simulink model "find6DOFSnellMin9_th"  (R2018b)
settings: Solver=ode8  StartTime=0.0  StopTime=length+1  FixedStep=1  RelTol=1e-3  EnableMultiTasking=on
StopFcn:
  | stopCallback
values from neighbouring files (symbols this model uses):
  botDot1 = zeros(length,2)    [find6DOFSnellMin9_ts.m]
  botDot2 = zeros(length,2)    [find6DOFSnellMin9_ts.m]
  botDot3 = zeros(length,2)    [find6DOFSnellMin9_ts.m]
libraries: find6DOFSnellMin9_cl x1
settings Model: SimulationMode=external  Creator=MAE-NCSUCORE  LastModifiedBy=MAE-NCSUCORE
settings SolverCC: ConcurrentTasks=on  AutoInsertRateTranBlk=on
settings DataIOCC: SaveFormat=StructureWithTime
settings OptimizationCC: BlockReduction=off  OptimizeBlockIOStorage=off  BufferReuse=off  GlobalBufferReuse=off  ExpressionFolding=off  LocalBlockOutputs=off  OptimizeDataStoreBuffers=off  BusAssignmentInplaceUpdate=off
settings DebuggingCC: UnitsInconsistencyMsg=none
settings HardwareCC: ProdBitPerPointer=32  ProdBitPerSizeT=32  ProdBitPerPtrDiffT=32  ProdLargestAtomicFloat=None  ProdWordSize=32  ProdLongLongMode=on  ProdHWDeviceType=Generic->32-bit x86 compatible
settings RTWCC: SystemTargetFile=slrt.tlc  TemplateMakefile=slrt_default_tmf  Description=Simulink Real-Time  CodeExecutionProfiling=on  RTWCompilerOptimization=on
settings SimulinkRealTimeCC: SupportVariableSizeSignals=on  PreserveStateflowLocalDataDimensions=off  RL32ObjectName=tg2  xPCisDefaultEnv=off  xPCTargetPCEnvName=Machine2  xPCConcurrentTasks=on

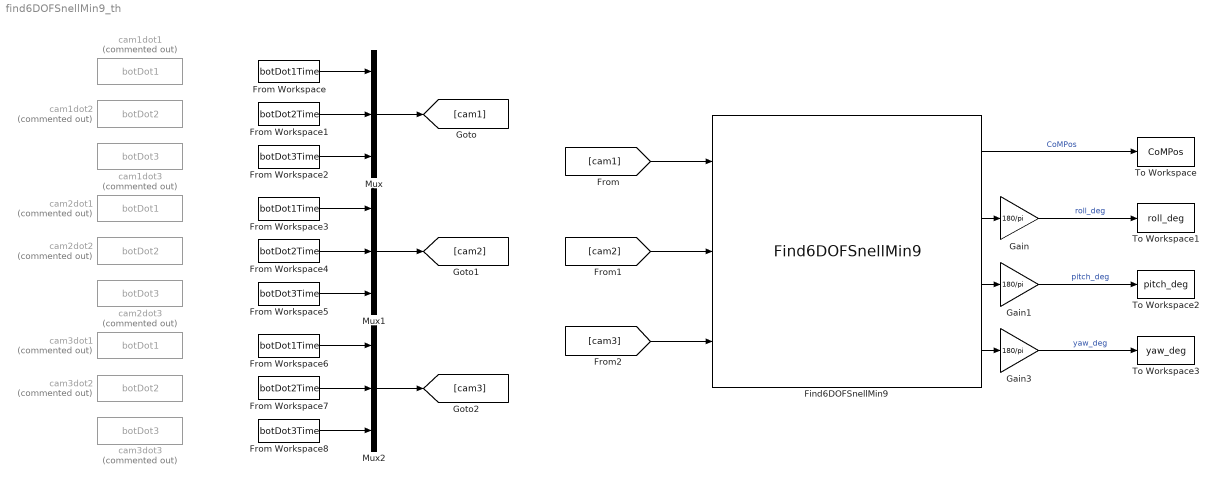
== system find6DOFSnellMin9_th ==
  Find6DOFSnellMin9 : find6DOFSnellMin9_cl/Find6DOFSnellMin9  imageDims_px=params.sideImageSize_px.Value  initialCoMPositionVec_cm=params.initCoMPosVec_cm.Value  initialEulerAngles_deg=params.initEulerAng_deg.Value  indxOfRefVec=params.indexOfRefractionA.Value  glassThickness_cm=params.glassThickness_cm.Value  snells=snells  cameraFOVAngles_deg=params.cameraFOV_deg.Value  sideEulerAngles_deg=params.sideCamEulAng_deg.Value  sideCamPositionVec_cm=params.sideCamPosVec_cm.Value  sideCamDistToGlass_cm=params.sideDistancetoGlass_cm.Value  botEulerAngles_deg=params.botCamEulAng_deg.Value  botCamPositionVec_cm=params.botCamPosVec_cm.Value  botCamDistToGlass_cm=params.botDistancetoGlass_cm.Value  slantEulerAngles_deg=params.slntCamEulAng_deg.Value  slantCamPositionVec_cm=params.slntCamPosVec_cm.Value  slantCamDistToGlass_cm=params.slntDistancetoGlass_cm.Value  sideSeparation_cm=params.sideDotSepDist_cm.Value  sidePositionVecBF_cm=params.sideDotPosVec_cm.Value  bottomASeparation_cm=params.botADotSepDist_cm.Value  botAPositionVecBF_cm=params.botADotPosVec_cm.Value  bottomBSeparation_cm=params.botBDotSepDist_cm.Value  botBPositionVecBF_cm=params.botBDotPosVec_cm.Value
  From Workspace : FromWorkspace  VariableName=botDot1Time  SampleTime=0
  From Workspace1 : FromWorkspace  VariableName=botDot2Time  SampleTime=0
  From Workspace2 : FromWorkspace  VariableName=botDot3Time  SampleTime=0
  From Workspace3 : FromWorkspace  VariableName=botDot1Time  SampleTime=0
  From Workspace4 : FromWorkspace  VariableName=botDot2Time  SampleTime=0
  From Workspace5 : FromWorkspace  VariableName=botDot3Time  SampleTime=0
  From Workspace6 : FromWorkspace  VariableName=botDot1Time  SampleTime=0
  From Workspace7 : FromWorkspace  VariableName=botDot2Time  SampleTime=0
  From Workspace8 : FromWorkspace  VariableName=botDot3Time  SampleTime=0
  Gain : Gain  Gain=180/pi
  Gain1 : Gain  Gain=180/pi
  Gain3 : Gain  Gain=180/pi
  Mux : Mux  Inputs=3
  Mux1 : Mux  Inputs=3
  Mux2 : Mux  Inputs=3
  To Workspace : ToWorkspace  VariableName=CoMPos  SaveFormat=Timeseries  SampleTime=-1
  To Workspace1 : ToWorkspace  VariableName=roll_deg  SaveFormat=Timeseries  SampleTime=-1
  To Workspace2 : ToWorkspace  VariableName=pitch_deg  SaveFormat=Timeseries  SampleTime=-1
  To Workspace3 : ToWorkspace  VariableName=yaw_deg  SaveFormat=Timeseries  SampleTime=-1
  cam1dot1 : Constant  Commented=on  Value=botDot1
  cam1dot2 : Constant  Commented=on  Value=botDot2
  cam1dot3 : Constant  Commented=on  Value=botDot3
  cam2dot1 : Constant  Commented=on  Value=botDot1
  cam2dot2 : Constant  Commented=on  Value=botDot2
  cam2dot3 : Constant  Commented=on  Value=botDot3
  cam3dot1 : Constant  Commented=on  Value=botDot1
  cam3dot2 : Constant  Commented=on  Value=botDot2
  cam3dot3 : Constant  Commented=on  Value=botDot3
  wires:
  Mux/1 -> [cam1]
  Mux2/1 -> [cam3]
  Mux1/1 -> [cam2]
  [cam1] -> Find6DOFSnellMin9/1
  [cam2] -> Find6DOFSnellMin9/2
  [cam3] -> Find6DOFSnellMin9/3
  Find6DOFSnellMin9/1 -> To Workspace/1  "CoMPos"
  Find6DOFSnellMin9/2 -> Gain/1
  Gain/1 -> To Workspace1/1  "roll_deg"
  Find6DOFSnellMin9/3 -> Gain1/1
  Gain1/1 -> To Workspace2/1  "pitch_deg"
  Find6DOFSnellMin9/4 -> Gain3/1
  Gain3/1 -> To Workspace3/1  "yaw_deg"
  From Workspace/1 -> Mux/1
  From Workspace1/1 -> Mux/2
  From Workspace2/1 -> Mux/3
  From Workspace6/1 -> Mux2/1
  From Workspace7/1 -> Mux2/2
  From Workspace8/1 -> Mux2/3
  From Workspace5/1 -> Mux1/3
  From Workspace4/1 -> Mux1/2
  From Workspace3/1 -> Mux1/1
